simulink model "PID"  (R2018a)
settings: Solver=VariableStepAuto  StartTime=0.0  StopTime=100  FixedStep=0.0001  MaxStep=1e-2  RelTol=1e-3  EnableMultiTasking=on
values from neighbouring files (symbols this model uses):
  C = (y_hat-y_ref)'*(y_hat-y_ref)/length(y_hat)    [QELandL.m]    (also in QEPID.m)
  Kc = K(1)    [QEPID.m]    (also in final_cube_alg.m = x(1))
  Td = 0    [QEPID.m]    (also in final_cube_alg.m = x(3))
  Ti = K(2)    [QEPID.m]    (also in final_cube_alg.m = x(2))
  w_o = K(3)    [QEPID.m]    (also in final_cube_alg.m = x(4))
  zeta_o = zeta    [QEPID.m]    (also in final_cube_alg.m = 0.9)
undefined symbols (not defined in the file or in its folder): A, B
libraries: simulink x4, slident x2, cstblocks x1
settings Model: Creator=rromano  LastModifiedBy=Marcelo
settings SolverCC: ZeroCrossAlgorithm=Adaptive  AutoInsertRateTranBlk=on
settings DataIOCC: LimitDataPoints=on  SaveFormat=Array  SignalLoggingSaveFormat=ModelDataLogs
settings OptimizationCC: ExpressionDepthLimit=2147483647  LifeSpan=inf
settings DebuggingCC: AlgebraicLoopMsg=none  UnderspecifiedInitializationDetection=Classic  MergeDetectMultiDrivingBlocksExec=none  MaxConsecutiveZCsMsg=none  SolverPrmCheckMsg=warning  FcnCallInpInsideContextMsg=warning  StateNameClashWarn=warning  SFUnexpectedBacktrackingDiag=warning  SFNoUnconditionalDefaultTransitionDiag=warning  SFExecutionAtInitializationDiag=none
settings HardwareCC: ProdBitPerPointer=32  ProdBitPerSizeT=32  ProdBitPerPtrDiffT=32  ProdLargestAtomicFloat=None  ProdIntDivRoundTo=Undefined  ProdEndianess=Unspecified  ProdWordSize=32  ProdHWDeviceType=32-bit Generic
settings ModelReferenceCC: PropagateSignalLabelsOutOfModel=off
settings CodeAppCC: StateflowObjectComments=on
settings GRTTargetCC: TargetLangStandard=C89/C90 (ANSI)  GeneratePreprocessorConditionals=Disable all  CombineOutputUpdateFcns=off  GRTInterface=on
settings ConfigComp: CovMetricSettings=dw  CovHtmlReporting=on  CovSaveCumulativeToWorkspaceVar=on  CovSaveSingleToWorkspaceVar=on  CovExternalEMLEnable=off

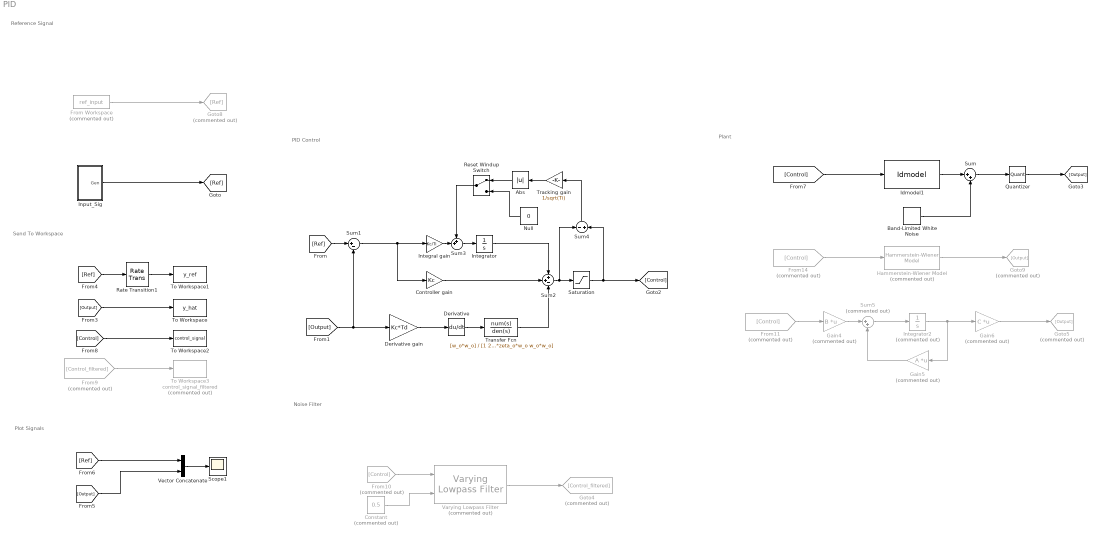
== system PID ==
  note: Noise Filter
  note: Plot Signals
  note: Send To Workspace
  note: Reference Signal
  note: PID Control
  note: Plant
  Abs : Abs
  Band-Limited White Noise : simulink/Sources/Band-Limited White Noise  Cov=[1e-04]  Ts=0.2  seed=[23341]
  Constant : Constant  Commented=on  Value=0.5
  Controller gain : Gain  Gain=Kc
  Derivative : Derivative
  Derivative gain : Gain  Gain=Kc*Td
  From Workspace : FromWorkspace  Commented=on  VariableName=ref_input  SampleTime=0
  From10 : From  Commented=on  GotoTag=Control
  From11 : From  Commented=on  GotoTag=Control
  From14 : From  Commented=on  GotoTag=Control
  From9 : From  Commented=on  GotoTag=Control_filtered
  Gain4 : Gain  Commented=on  Gain=B  Multiplication=Matrix(K*u)
  Gain5 : Gain  Commented=on  Gain=A  Multiplication=Matrix(K*u)
  Gain6 : Gain  Commented=on  Gain=C  Multiplication=Matrix(K*u)
  Goto4 : Goto  Commented=on  GotoTag=Control_filtered
  Goto5 : Goto  Commented=on  GotoTag=Output
  Goto8 : Goto  Commented=on  GotoTag=Ref
  Goto9 : Goto  Commented=on  GotoTag=Output
  Hammerstein-Wiener Model : slident/Models/Hammerstein-Wiener Model  Commented=on  sys=linear_app  IC=Zero  X0i=0
      settings: SourceProductName=System Identification Toolbox  SourceProductBaseCode=ID
  Idmodel1 : slident/Models/Idmodel  sys=linear_app  IC=0  noi=off  seed=[]
      settings: SourceProductName=System Identification Toolbox  SourceProductBaseCode=ID
  Input_Sig : Subsystem
  Integral gain : Gain  Gain=Kc/Ti
  Integrator : Integrator  ZeroCross=off
  Integrator2 : Integrator  Commented=on  ZeroCross=off
  Null : Constant  Value=0
  Quantizer : Quantizer  QuantizationInterval=0.3516
  Rate Transition1 : RateTransition  OutPortSampleTime=0.2
  Reset Windup Switch : ManualSwitch
  Saturation : Saturate  UpperLimit=5000  LowerLimit=-5000  ZeroCross=off
  Scope1 : Scope
  Sum : Sum  Inputs=|++
  Sum1 : Sum  Inputs=|+-
  Sum2 : Sum  Inputs=++-
  Sum3 : Sum  Inputs=++|
  Sum4 : Sum  Inputs=-|+
  Sum5 : Sum  Commented=on  Inputs=|++
  To Workspace : ToWorkspace  VariableName=y_hat  SampleTime=-1
      settings: Save2DSignal=2-D array (concatenate along first dimension)
  To Workspace1 : ToWorkspace  VariableName=y_ref  SampleTime=-1
      settings: Save2DSignal=2-D array (concatenate along first dimension)
  To Workspace2 : ToWorkspace  VariableName=control_signal  SampleTime=-1
      settings: Save2DSignal=2-D array (concatenate along first dimension)
  To Workspace3 : ToWorkspace  Commented=on  VariableName=control_signal_filtered  SaveFormat=Timeseries  SampleTime=-1
      settings: Save2DSignal=2-D array (concatenate along first dimension)
  Tracking gain : Gain  Gain=1/sqrt(Ti)
  Transfer Fcn : TransferFcn  Numerator=[w_o*w_o]  Denominator=[1 2*zeta_o*w_o w_o*w_o]
  Varying Lowpass Filter : cstblocks/Linear Parameter Varying/Varying Lowpass Filter  Commented=on  N=1
      settings: SourceProductName=Control System Toolbox
  Vector Concatenate : Concatenate
  wires:
  Vector Concatenate/1 -> Scope1/1
  Reset Windup Switch/1 -> Sum3/1
  Tracking gain/1 -> Abs/1
  Null/1 -> Reset Windup Switch/2
  Controller gain/1 -> Sum2/2
  Derivative gain/1 -> Derivative/1
  Sum3/1 -> Integrator/1
  Saturation/1 -> [Control], Sum4/2
  Sum2/1 -> Sum4/1, Saturation/1
  Integrator/1 -> Sum2/1
  Integral gain/1 -> Sum3/2
  [Ref] -> Sum1/1
  Sum1/1 -> Controller gain/1, Integral gain/1
  [Output] -> To Workspace/1
  [Ref] -> Rate Transition1/1
  [Ref] -> Vector Concatenate/1
  [Output] -> Vector Concatenate/2
  [Control] -> Idmodel1/1
  [Output] -> Derivative gain/1, Sum1/2
  [Control] -> To Workspace2/1
  From9/1 -> To Workspace3/1
  From10/1 -> Varying Lowpass Filter/1
  Constant/1 -> Varying Lowpass Filter/2
  Varying Lowpass Filter/1 -> Goto4/1
  Gain6/1 -> Goto5/1
  From11/1 -> Gain4/1
  Gain4/1 -> Sum5/1
  Sum5/1 -> Integrator2/1
  Gain5/1 -> Sum5/2
  Integrator2/1 -> Gain5/1, Gain6/1
  Sum4/1 -> Tracking gain/1
  Derivative/1 -> Transfer Fcn/1
  Transfer Fcn/1 -> Sum2/3
  Rate Transition1/1 -> To Workspace1/1
  From Workspace/1 -> Goto8/1
  Hammerstein-Wiener Model/1 -> Goto9/1
  From14/1 -> Hammerstein-Wiener Model/1
  Input_Sig/1(Gen) -> [Ref]
  Abs/1 -> Reset Windup Switch/1
  Idmodel1/1 -> Sum/1
  Band-Limited White Noise/1 -> Sum/2
  Sum/1 -> Quantizer/1
  Quantizer/1 -> [Output]

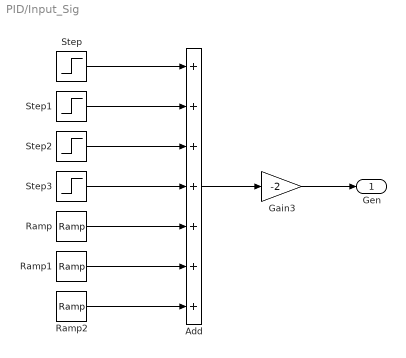
== system PID/Input_Sig ==
  Add : Sum  Inputs=+++++++
  Gain3 : Gain  Gain=-2
  Ramp : simulink/Sources/Ramp  slope=2  start=70  InitialOutput=0
  Ramp1 : simulink/Sources/Ramp  slope=-4  start=80  InitialOutput=0
  Ramp2 : simulink/Sources/Ramp  slope=2  start=90  InitialOutput=0
  Step : Step  Time=5  After=10  SampleTime=0
  Step1 : Step  Time=25  After=-20  SampleTime=0
  Step2 : Step  Time=35  After=35  SampleTime=0
  Step3 : Step  Time=50  After=-25  SampleTime=0
  Gen : Outport
  wires:
  Ramp1/1 -> Add/6
  Ramp2/1 -> Add/7
  Step3/1 -> Add/4
  Step2/1 -> Add/3
  Ramp/1 -> Add/5
  Add/1 -> Gain3/1
  Step1/1 -> Add/2
  Step/1 -> Add/1
  Gain3/1 -> Gen/1
